simulink model "FastAgc"  (R2016a)
settings: Solver=VariableStepAuto  StartTime=0.0  StopTime=0.0003  RelTol=1e-3
undefined symbols (not defined in the file or in its folder): Br, RC, Ts
libraries: xbsIndex_r4 x45, commchan3 x1, commdigbbndpm3 x1, dspsrcs4 x1, dspfdesign x1, commrandsrc3 x1, simulink x1
settings Model: Creator=frank  LastModifiedBy=frank

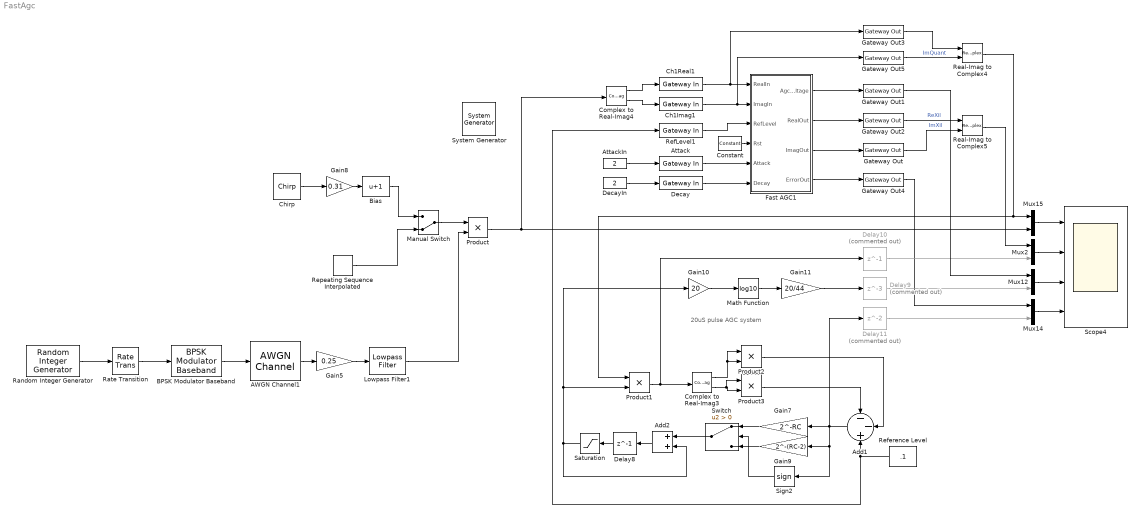
== system FastAgc ==
  note: 20uS pulse AGC system
  " System Generator" : xbsIndex_r4/ System Generator  Tag=genX  xilinxfamily=kintex7  part=xc7k325t  speed=-2  package=fbg676  synthesis_tool=Vivado  clock_wrapper=Clock Enables  directory=./netlist  proj_type=Vivado  Synth_file=Vivado Synthesis Defaults  Impl_file=Vivado Implementation Defaults  testbench=off  simulink_period=Ts  sysclk_period=3000/280  dcm_input_clock_period=10  incr_netlist=off  trim_vbits=Everywhere in SubSystem  dbl_ovrd=According to Block Masks  core_generation=According to Block Masks  run_coregen=off  deprecated_control=off  eval_field=0  block_type=sysgen
  AWGN Channel1 : commchan3/AWGN Channel  InputProcessing=Columns as channels (frame based)  seed=67  noiseMode="Signal to noise ratio  (Eb/No)"  EbNodB=EbNo  EsNodB=10  SNRdB=10  bitsPerSym=2  Ps=1  Tsym=1/Br  variance=1
  Add1 : Sum  Inputs=--+  OutDataTypeStr=Inherit: Same as first input
  Add2 : Sum
  Attack : xbsIndex_r4/Gateway In  gui_display_data_type=Fixed-point  arith_type=Unsigned  n_bits=3  bin_pt=0  preci_type=Single  exp_width=8  frac_width=24  rows=1  columns=1  quantization="Round  (unbiased: +/- Inf)"  overflow=Saturate  period=Ts  UseAsADC=off  ADCChannel='1'  interface=None  automatic_assignment=on  address_offset=hex2dec('00')  intf_name=''  intf_description=''  default_value=0  timing_constraint=None  locs_specified=off  LOCs={}  io_standard={}  inherit_from_input=off  hdl_port=on  dbl_ovrd=off  block_type=gatewayin
  AttackIn : Constant  Value=2
  BPSK Modulator Baseband : commdigbbndpm3/BPSK Modulator Baseband  Ph=0  outDtype=double  outWordLen=16  outUDDataType=sfix(16)  outFracLenMode=Best precision  outFracLen=15  outDataTypeStr=double  outLastDataTypeStr=double
  Bias : Bias  Bias=1
  Ch1Imag1 : xbsIndex_r4/Gateway In  gui_display_data_type=Fixed-point  arith_type="Signed  (2's comp)"  n_bits=18  bin_pt=17  preci_type=Single  exp_width=8  frac_width=24  rows=1  columns=1  quantization="Round  (unbiased: +/- Inf)"  overflow=Saturate  period=Ts  UseAsADC=off  ADCChannel='1'  interface=None  automatic_assignment=on  address_offset=hex2dec('00')  intf_name=''  intf_description=''  default_value=0  timing_constraint=None  locs_specified=off  LOCs={}  io_standard={}  inherit_from_input=off  hdl_port=on  dbl_ovrd=off  block_type=gatewayin
  Ch1Real1 : xbsIndex_r4/Gateway In  gui_display_data_type=Fixed-point  arith_type="Signed  (2's comp)"  n_bits=18  bin_pt=17  preci_type=Single  exp_width=8  frac_width=24  rows=1  columns=1  quantization="Round  (unbiased: +/- Inf)"  overflow=Saturate  period=Ts  UseAsADC=off  ADCChannel='1'  interface=None  automatic_assignment=on  address_offset=hex2dec('00')  intf_name=''  intf_description=''  default_value=0  timing_constraint=None  locs_specified=off  LOCs={}  io_standard={}  inherit_from_input=off  hdl_port=on  dbl_ovrd=off  block_type=gatewayin
  Chirp : dspsrcs4/Chirp  sweep=Logarithmic  mode=Unidirectional  f0=1000  f1=100000  t1=0.01  Tsweep=0.01  phase=0  Ts=Ts  spf=1  datatype=Double  OutputFrames=off
  Complex to Real-Imag3 : ComplexToRealImag
  Complex to Real-Imag4 : ComplexToRealImag
  Constant : xbsIndex_r4/Constant  const=0  gui_display_data_type=Boolean  arith_type=Boolean  n_bits=16  bin_pt=14  preci_type=Single  exp_width=8  frac_width=24  explicit_period=off  period=1  equ=P=C  opselect=C  inp2=PCIN>>17  opr=+  inp1=P  carry=CIN  dbl_ovrd=off  block_type=constant
  Decay : xbsIndex_r4/Gateway In  gui_display_data_type=Fixed-point  arith_type=Unsigned  n_bits=3  bin_pt=0  preci_type=Single  exp_width=8  frac_width=24  rows=1  columns=1  quantization="Round  (unbiased: +/- Inf)"  overflow=Saturate  period=Ts  UseAsADC=off  ADCChannel='1'  interface=None  automatic_assignment=on  address_offset=hex2dec('00')  intf_name=''  intf_description=''  default_value=0  timing_constraint=None  locs_specified=off  LOCs={}  io_standard={}  inherit_from_input=off  hdl_port=on  dbl_ovrd=off  block_type=gatewayin
  DecayIn : Constant  Value=2
  Delay10 : Delay  Commented=on  DelayLength=1
  Delay11 : Delay  Commented=on
  Delay8 : Delay  DelayLength=1
  Delay9 : Delay  Commented=on  DelayLength=3
  Fast AGC1 : Subsystem
  Gain10 : Gain  Gain=20
  Gain11 : Gain  Gain=20/44
  Gain5 : Gain  Gain=0.25
  Gain7 : Gain  Gain=2^-RC
  Gain8 : Gain  Gain=0.31
  Gain9 : Gain  Gain=2^-(RC-2)
  Gateway Out{,1..5} (6 alike) : xbsIndex_r4/Gateway Out  inherit_from_input=off  hdl_port=on  rows=1  columns=1  UseAsDAC=off  DACChannel='1'  interface=None  automatic_assignment=on  address_offset=hex2dec('00')  intf_name=''  intf_description=''  timing_constraint=None  locs_specified=off  LOCs={}  io_standard={}  block_type=gatewayout
  Lowpass Filter1 : dspfdesign/Lowpass Filter  FilterType=FIR  DesignForMinimumOrder=on  FilterOrder=50  PassbandFrequency=Br/2  StopbandFrequency=Br*2  PassbandRipple=0.1  StopbandAttenuation=80  InheritSampleRate=off  SampleRate=1/Ts  roundingMode=Floor  coeffsDataTypeStr=fixdt(1,16)  SimulateUsing=Interpreted execution
  Manual Switch : ManualSwitch  CurrentSetting=0
  Math Function : Math  Operator=log10  SaturateOnIntegerOverflow=on
  Mux{2,12,14..15} (4 alike) : Mux  Inputs=2
  Product{,1..3} (4 alike) : Product
  Random Integer Generator : commrandsrc3/Random Integer Generator  SetSize=2  SeedSource=Auto  Seed=0  SampleTime=1/Br  SamplesPerFrame=1  OutputDataType=double  SimulateUsing=Code generation
  Rate Transition : RateTransition  OutPortSampleTime=Ts
  Real-Imag to Complex4 : RealImagToComplex
  Real-Imag to Complex5 : RealImagToComplex
  RefLevel1 : xbsIndex_r4/Gateway In  gui_display_data_type=Fixed-point  arith_type=Unsigned  n_bits=18  bin_pt=17  preci_type=Single  exp_width=8  frac_width=24  rows=1  columns=1  quantization="Round  (unbiased: +/- Inf)"  overflow=Saturate  period=Ts  UseAsADC=off  ADCChannel='1'  interface=None  automatic_assignment=on  address_offset=hex2dec('00')  intf_name=''  intf_description=''  default_value=0  timing_constraint=None  locs_specified=off  LOCs={}  io_standard={}  inherit_from_input=off  hdl_port=on  dbl_ovrd=off  block_type=gatewayin
  Reference Level : Constant  Value=.1
  Repeating Sequence Interpolated : simulink/Sources/Repeating Sequence Interpolated  OutValues=[10 1 .01 .01 10 10].'  TimeValues=[0 2e-5 3e-5 14e-5 15e-5 2e-4].'  LookUpMeth=Interpolation-Use End Values  tsamp=Ts  OutMin=[]  OutMax=[]  OutDataTypeStr=double  OutputDataTypeScalingMode=double  OutDataType=fixdt(0,8)  OutScaling=2^-10
  Saturation : Saturate  UpperLimit=15  LowerLimit=0.5
  Scope4 : Scope  NumInputPorts=4
  Sign2 : Signum
  Switch : Switch  Criteria=u2 > Threshold
  wires:
  Lowpass Filter1/1 -> Product/2
  Add2/1 -> Delay8/1
  Complex to Real-Imag3/2 -> Product3/1, Product3/2
  Complex to Real-Imag3/1 -> Product2/1, Product2/2
  Add1/1 -> Delay11/1, Gain7/1, Sign2/1, Gain9/1
  Product3/1 -> Add1/1
  Product2/1 -> Add1/2
  Reference Level/1 -> Add1/3, RefLevel1/1
  Manual Switch/1 -> Product/1
  Repeating Sequence Interpolated/1 -> Manual Switch/2
  Switch/1 -> Add2/1
  Gain7/1 -> Switch/1
  Gain9/1 -> Switch/3
  Sign2/1 -> Switch/2
  Delay8/1 -> Saturation/1
  Chirp/1 -> Gain8/1
  Ch1Real1/1 -> Gateway Out3/1, Fast AGC1/1(RealIn)
  Gateway Out2/1 -> Real-Imag to Complex5/1  "ReXil"
  Gateway Out/1 -> Real-Imag to Complex5/2  "ImXil"
  Complex to Real-Imag4/1 -> Ch1Real1/1
  Complex to Real-Imag4/2 -> Ch1Imag1/1
  Ch1Imag1/1 -> Gateway Out5/1, Fast AGC1/2(ImagIn)
  Fast AGC1/1(AgcVoltage) -> Gateway Out1/1
  Fast AGC1/2(RealOut) -> Gateway Out2/1
  Fast AGC1/3(ImagOut) -> Gateway Out/1
  RefLevel1/1 -> Fast AGC1/3(RefLevel)
  Real-Imag to Complex5/1 -> Mux2/1
  Fast AGC1/4(ErrorOut) -> Gateway Out4/1
  Gateway Out4/1 -> Mux14/1
  Gateway Out5/1 -> Real-Imag to Complex4/2  "ImQuant"
  Delay10/1 -> Mux2/2
  Delay9/1 -> Mux12/2
  Delay11/1 -> Mux14/2
  Gain8/1 -> Bias/1
  Product/1 -> Mux15/2, Complex to Real-Imag4/1
  Real-Imag to Complex4/1 -> Mux15/1, Product1/1
  Math Function/1 -> Gain11/1
  Saturation/1 -> Add2/2, Gain10/1, Product1/2
  Gain10/1 -> Math Function/1
  Gateway Out1/1 -> Mux12/1
  Gain11/1 -> Delay9/1
  Product1/1 -> Delay10/1, Complex to Real-Imag3/1
  Bias/1 -> Manual Switch/1
  Mux15/1 -> Scope4/1
  Mux2/1 -> Scope4/2
  Mux12/1 -> Scope4/3
  Mux14/1 -> Scope4/4
  Constant/1 -> Fast AGC1/4(Rst)
  Random Integer Generator/1 -> Rate Transition/1
  Rate Transition/1 -> BPSK Modulator Baseband/1
  BPSK Modulator Baseband/1 -> AWGN Channel1/1
  AWGN Channel1/1 -> Gain5/1
  Gain5/1 -> Lowpass Filter1/1
  Gateway Out3/1 -> Real-Imag to Complex4/1
  Attack/1 -> Fast AGC1/5(Attack)
  Decay/1 -> Fast AGC1/6(Decay)
  AttackIn/1 -> Attack/1
  DecayIn/1 -> Decay/1

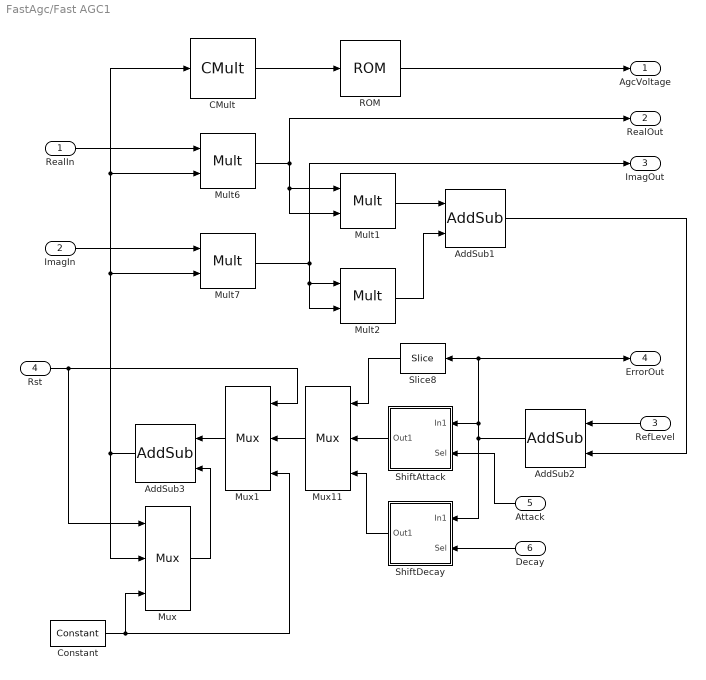
== system FastAgc/Fast AGC1 ==
  RealIn : Inport
  ImagIn : Inport  Port=2
  RefLevel : Inport  Port=3
  Rst : Inport  Port=4
  Attack : Inport  Port=5
  Decay : Inport  Port=6
  AddSub1 : xbsIndex_r4/AddSub  mode=Addition  use_carryin=off  use_carryout=off  en=off  latency=0  precision=Full  arith_type=Unsigned  n_bits=18  bin_pt=18  quantization=Truncate  overflow=Saturate  use_behavioral_HDL=off  hw_selection=Fabric  pipelined=off  dbl_ovrd=off  block_type=addsub
  AddSub2 : xbsIndex_r4/AddSub  mode=Subtraction  use_carryin=off  use_carryout=off  en=off  latency=1  precision=Full  arith_type=Unsigned  n_bits=18  bin_pt=18  quantization=Truncate  overflow=Saturate  use_behavioral_HDL=off  hw_selection=Fabric  pipelined=off  dbl_ovrd=off  block_type=addsub
  AddSub3 : xbsIndex_r4/AddSub  mode=Addition  use_carryin=off  use_carryout=off  en=off  latency=1  precision=User Defined  arith_type=Unsigned  n_bits=18  bin_pt=13  quantization=Truncate  overflow=Saturate  use_behavioral_HDL=off  hw_selection=Fabric  pipelined=off  dbl_ovrd=off  block_type=addsub
  CMult : xbsIndex_r4/CMult  const=64  gui_display_data_type=Fixed-point  const_n_bits=7  const_bin_pt=0  float_type=Single  exp_bits=8  fraction_bits=24  en=off  latency=0  precision=User Defined  arith_type=Unsigned  n_bits=10  bin_pt=0  quantization=Truncate  overflow=Saturate  use_behavioral_HDL=off  mem_type=Distributed RAM  pipeline=off  dbl_ovrd=off  block_type=cmult
  Constant : xbsIndex_r4/Constant  const=0  gui_display_data_type=Fixed-point  arith_type=Unsigned  n_bits=18  bin_pt=13  preci_type=Single  exp_width=8  frac_width=24  explicit_period=on  period=Ts  equ=P=C  opselect=C  inp2=PCIN>>17  opr=+  inp1=P  carry=CIN  dbl_ovrd=off  block_type=constant
  Mult1 : xbsIndex_r4/Mult  precision=User Defined  arith_type=Unsigned  n_bits=18  bin_pt=17  quantization=Truncate  overflow=Wrap  en=off  latency=1  use_behavioral_HDL=off  opt=Speed  use_embedded=on  optimum_pipeline=off  pipeline=on  dbl_ovrd=off  use_rpm=on  placement_style=Triangular  block_type=mult
  Mult2 : xbsIndex_r4/Mult  precision=User Defined  arith_type=Unsigned  n_bits=18  bin_pt=17  quantization=Truncate  overflow=Wrap  en=off  latency=1  use_behavioral_HDL=off  opt=Speed  use_embedded=on  optimum_pipeline=off  pipeline=on  dbl_ovrd=off  use_rpm=on  placement_style=Triangular  block_type=mult
  Mult6 : xbsIndex_r4/Mult  precision=User Defined  arith_type="Signed  (2's comp)"  n_bits=18  bin_pt=17  quantization=Truncate  overflow=Saturate  en=off  latency=1  use_behavioral_HDL=off  opt=Speed  use_embedded=on  optimum_pipeline=off  pipeline=on  dbl_ovrd=off  use_rpm=on  placement_style=Triangular  block_type=mult
  Mult7 : xbsIndex_r4/Mult  precision=User Defined  arith_type="Signed  (2's comp)"  n_bits=18  bin_pt=17  quantization=Truncate  overflow=Saturate  en=off  latency=1  use_behavioral_HDL=off  opt=Speed  use_embedded=on  optimum_pipeline=off  pipeline=on  dbl_ovrd=off  use_rpm=on  placement_style=Triangular  block_type=mult
  Mux : xbsIndex_r4/Mux  inputs=2  en=off  latency=0  precision=Full  arith_type=Unsigned  n_bits=16  bin_pt=14  quantization=Truncate  overflow=Wrap  dbl_ovrd=off  block_type=mux
  Mux1 : xbsIndex_r4/Mux  inputs=2  en=off  latency=0  precision=Full  arith_type=Unsigned  n_bits=16  bin_pt=14  quantization=Truncate  overflow=Wrap  dbl_ovrd=off  block_type=mux
  Mux11 : xbsIndex_r4/Mux  inputs=2  en=off  latency=0  precision=Full  arith_type=Unsigned  n_bits=16  bin_pt=14  quantization=Truncate  overflow=Wrap  dbl_ovrd=off  block_type=mux
  ROM : xbsIndex_r4/ROM  depth=1024  initVector=[log10((0:1023)/64)]/44  distributed_mem=Block RAM  rst=off  init_reg=0  en=off  latency=1  gui_display_data_type=Fixed-point  arith_type=Unsigned  n_bits=18  bin_pt=17  preci_type=Single  exp_width=8  frac_width=24  optimize=Area  use_rpm=on  dbl_ovrd=off  block_type=sprom
  ShiftAttack : Subsystem
  ShiftDecay : Subsystem
  Slice8 : xbsIndex_r4/Slice  nbits=1  boolean_output=on  mode=Upper Bit Location + Width  bit1=0  base1=MSB of Input  bit0=0  base0=LSB of Input  dbl_ovrd=off  block_type=slice
  AgcVoltage : Outport
  RealOut : Outport  Port=2
  ImagOut : Outport  Port=3
  ErrorOut : Outport  Port=4
  wires:
  Constant/1 -> Mux1/3, Mux/3
  Decay/1 -> ShiftDecay/2(Sel)
  Attack/1 -> ShiftAttack/2(Sel)
  ShiftAttack/1(Out1) -> Mux11/2
  AddSub3/1 -> Mult7/2, CMult/1, Mult6/2, Mux/2
  AddSub1/1 -> AddSub2/2
  RealIn/1 -> Mult6/1
  RefLevel/1 -> AddSub2/1
  Mult7/1 -> Mult2/2, Mult2/1, ImagOut/1
  Mult6/1 -> Mult1/1, Mult1/2, RealOut/1
  Mult1/1 -> AddSub1/1
  ImagIn/1 -> Mult7/1
  Mult2/1 -> AddSub1/2
  AddSub2/1 -> Slice8/1, ErrorOut/1, ShiftAttack/1(In1), ShiftDecay/1(In1)
  ShiftDecay/1(Out1) -> Mux11/3
  Mux11/1 -> Mux1/2
  Slice8/1 -> Mux11/1
  CMult/1 -> ROM/1
  ROM/1 -> AgcVoltage/1
  Mux/1 -> AddSub3/2
  Rst/1 -> Mux1/1, Mux/1
  Mux1/1 -> AddSub3/1

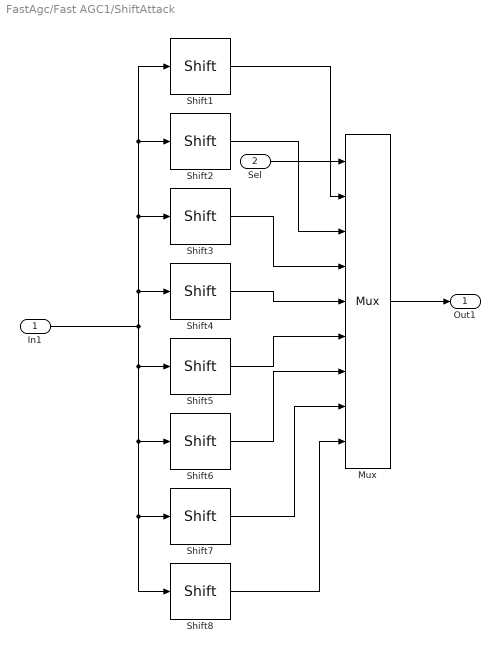
== system FastAgc/Fast AGC1/ShiftAttack ==
  In1 : Inport
  Sel : Inport  Port=2
  Mux : xbsIndex_r4/Mux  inputs=8  en=off  latency=0  precision=Full  arith_type=Unsigned  n_bits=16  bin_pt=14  quantization=Truncate  overflow=Wrap  dbl_ovrd=off  block_type=mux
  Shift1 : xbsIndex_r4/Shift  shift_dir=Right  shift_bits=1  en=off  latency=0  precision=Full  arith_type="Signed  (2's comp)"  n_bits=16  bin_pt=14  quantization=Truncate  overflow=Wrap  dbl_ovrd=off  block_type=shift
  Shift2 : xbsIndex_r4/Shift  shift_dir=Right  shift_bits=2  en=off  latency=0  precision=Full  arith_type="Signed  (2's comp)"  n_bits=16  bin_pt=14  quantization=Truncate  overflow=Wrap  dbl_ovrd=off  block_type=shift
  Shift3 : xbsIndex_r4/Shift  shift_dir=Right  shift_bits=3  en=off  latency=0  precision=Full  arith_type="Signed  (2's comp)"  n_bits=16  bin_pt=14  quantization=Truncate  overflow=Wrap  dbl_ovrd=off  block_type=shift
  Shift4 : xbsIndex_r4/Shift  shift_dir=Right  shift_bits=4  en=off  latency=0  precision=Full  arith_type="Signed  (2's comp)"  n_bits=16  bin_pt=14  quantization=Truncate  overflow=Wrap  dbl_ovrd=off  block_type=shift
  Shift5 : xbsIndex_r4/Shift  shift_dir=Right  shift_bits=5  en=off  latency=0  precision=Full  arith_type="Signed  (2's comp)"  n_bits=16  bin_pt=14  quantization=Truncate  overflow=Wrap  dbl_ovrd=off  block_type=shift
  Shift6 : xbsIndex_r4/Shift  shift_dir=Right  shift_bits=6  en=off  latency=0  precision=Full  arith_type="Signed  (2's comp)"  n_bits=16  bin_pt=14  quantization=Truncate  overflow=Wrap  dbl_ovrd=off  block_type=shift
  Shift7 : xbsIndex_r4/Shift  shift_dir=Right  shift_bits=7  en=off  latency=0  precision=Full  arith_type="Signed  (2's comp)"  n_bits=16  bin_pt=14  quantization=Truncate  overflow=Wrap  dbl_ovrd=off  block_type=shift
  Shift8 : xbsIndex_r4/Shift  shift_dir=Right  shift_bits=8  en=off  latency=0  precision=Full  arith_type="Signed  (2's comp)"  n_bits=16  bin_pt=14  quantization=Truncate  overflow=Wrap  dbl_ovrd=off  block_type=shift
  Out1 : Outport
  wires:
  Sel/1 -> Mux/1
  Mux/1 -> Out1/1
  Shift8/1 -> Mux/9
  Shift7/1 -> Mux/8
  Shift2/1 -> Mux/3
  Shift6/1 -> Mux/7
  Shift3/1 -> Mux/4
  Shift5/1 -> Mux/6
  Shift4/1 -> Mux/5
  In1/1 -> Shift8/1, Shift7/1, Shift6/1, Shift5/1, Shift1/1, Shift2/1, Shift3/1, Shift4/1
  Shift1/1 -> Mux/2

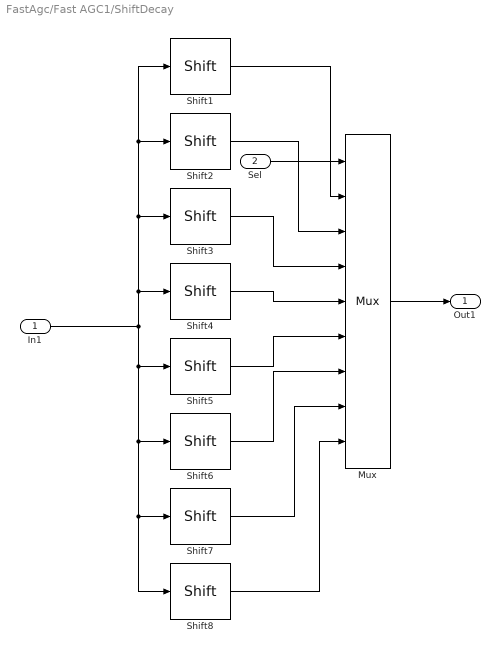
== system FastAgc/Fast AGC1/ShiftDecay ==
  In1 : Inport
  Sel : Inport  Port=2
  Mux : xbsIndex_r4/Mux  inputs=8  en=off  latency=0  precision=Full  arith_type=Unsigned  n_bits=16  bin_pt=14  quantization=Truncate  overflow=Wrap  dbl_ovrd=off  block_type=mux
  Shift1 : xbsIndex_r4/Shift  shift_dir=Right  shift_bits=1  en=off  latency=0  precision=Full  arith_type="Signed  (2's comp)"  n_bits=16  bin_pt=14  quantization=Truncate  overflow=Wrap  dbl_ovrd=off  block_type=shift
  Shift2 : xbsIndex_r4/Shift  shift_dir=Right  shift_bits=2  en=off  latency=0  precision=Full  arith_type="Signed  (2's comp)"  n_bits=16  bin_pt=14  quantization=Truncate  overflow=Wrap  dbl_ovrd=off  block_type=shift
  Shift3 : xbsIndex_r4/Shift  shift_dir=Right  shift_bits=3  en=off  latency=0  precision=Full  arith_type="Signed  (2's comp)"  n_bits=16  bin_pt=14  quantization=Truncate  overflow=Wrap  dbl_ovrd=off  block_type=shift
  Shift4 : xbsIndex_r4/Shift  shift_dir=Right  shift_bits=4  en=off  latency=0  precision=Full  arith_type="Signed  (2's comp)"  n_bits=16  bin_pt=14  quantization=Truncate  overflow=Wrap  dbl_ovrd=off  block_type=shift
  Shift5 : xbsIndex_r4/Shift  shift_dir=Right  shift_bits=5  en=off  latency=0  precision=Full  arith_type="Signed  (2's comp)"  n_bits=16  bin_pt=14  quantization=Truncate  overflow=Wrap  dbl_ovrd=off  block_type=shift
  Shift6 : xbsIndex_r4/Shift  shift_dir=Right  shift_bits=6  en=off  latency=0  precision=Full  arith_type="Signed  (2's comp)"  n_bits=16  bin_pt=14  quantization=Truncate  overflow=Wrap  dbl_ovrd=off  block_type=shift
  Shift7 : xbsIndex_r4/Shift  shift_dir=Right  shift_bits=7  en=off  latency=0  precision=Full  arith_type="Signed  (2's comp)"  n_bits=16  bin_pt=14  quantization=Truncate  overflow=Wrap  dbl_ovrd=off  block_type=shift
  Shift8 : xbsIndex_r4/Shift  shift_dir=Right  shift_bits=8  en=off  latency=0  precision=Full  arith_type="Signed  (2's comp)"  n_bits=16  bin_pt=14  quantization=Truncate  overflow=Wrap  dbl_ovrd=off  block_type=shift
  Out1 : Outport
  wires:
  Shift1/1 -> Mux/2
  In1/1 -> Shift4/1, Shift3/1, Shift2/1, Shift1/1, Shift5/1, Shift6/1, Shift7/1, Shift8/1
  Shift4/1 -> Mux/5
  Shift5/1 -> Mux/6
  Shift3/1 -> Mux/4
  Shift6/1 -> Mux/7
  Shift2/1 -> Mux/3
  Shift7/1 -> Mux/8
  Shift8/1 -> Mux/9
  Mux/1 -> Out1/1
  Sel/1 -> Mux/1
